simulink model "MyBattery_RTW"  (Simulink 8.5)
settings: Solver=ode1  SolverMode=SingleTasking  StartTime=0.0  StopTime=inf  FixedStep=0.0002  RelTol=1e-3
PreLoadFcn:
  | vehicle = 'Car'; if ~length(which('cmcmd')), cmenv; end
  | MyBattery_RTW_bus
InitFcn:
  | vehicle = 'Car'; if ~length(which('cmcmd')), cmenv; end
  | MyBattery_RTW_bus
libraries: CarMaker4SL x2, simulink x2
Description:
  | CarMaker Real-Time Target (64-bit)
settings Model: Creator=ml  LastModifiedBy=ml
settings DebuggingCC: FcnCallInpInsideContextMsg=UseLocalSettings
settings HardwareCC: TargetHWDeviceType=32-bit Generic  ProdEqTarget=off
settings RTWCC: SystemTargetFile=CarMaker64.tlc  TemplateMakefile=CarMaker_unix64.tmf  Description=CarMaker Real-Time Target (64-bit)
settings CodeAppCC: MaxIdLength=63
settings STFCustomTargetCC: ModelReferenceCompliant=off  GeneratePreprocessorConditionals=Disable all  MultiInstanceERTCode=on  CodeInterfacePackaging=Reusable function  CPPClassGenCompliant=on  GRTInterface=off  GenerateAllocFcn=on  SystemTargetFile=CarMaker64.tlc
settings GRTTargetCC: ModelReferenceCompliant=off  ParMdlRefBuildCompliant=off  CompOptLevelCompliant=off  ConcurrentExecutionCompliant=off  MatFileLogging=off  MultiInstanceERTCode=on  CodeInterfacePackaging=Reusable function  GRTInterface=off  GenerateAllocFcn=on  ExtModeMexFile=noextcomm
settings CustomProperty: DataType=string  Value=..
settings EnumStrPairs: String=Car

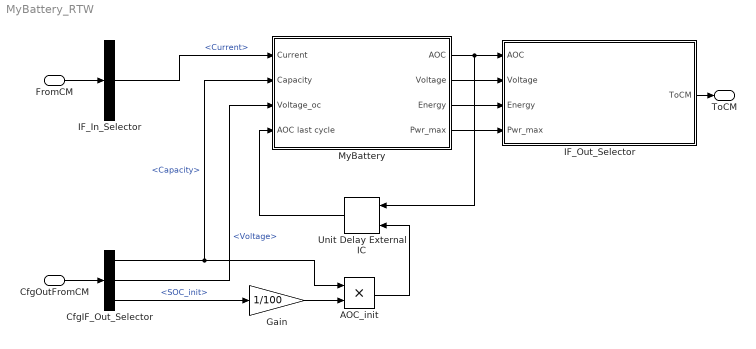
== system MyBattery_RTW ==
  FromCM : Inport  OutDataTypeStr=Bus: cmPTBatteryIn
  CfgOutFromCM : Inport  Port=2  OutDataTypeStr=Bus: cmPTBatteryCfgOut
  AOC_init : Product  RndMeth=Zero
  CfgIF_Out_Selector : BusSelector  OutputSignals=Capacity,Voltage,SOC_init
  Gain : Gain  Gain=1/100
  IF_In_Selector : BusSelector  OutputSignals=Current
  IF_Out_Selector : Subsystem  mask(Signal Selection){}
      mask help: Signal Selection Block
      settings: OpenFcn=cmSignalSelect('SignalSelection_CB',gcb)
  MyBattery : Subsystem
  Unit Delay External IC : simulink/Additional Math & Discrete/Additional Discrete/Unit Delay External IC  tsamp=-1
  ToCM : Outport  OutDataTypeStr=Bus: cmPTBatteryOut
  wires:
  FromCM/1 -> IF_In_Selector/1
  IF_Out_Selector/1(ToCM) -> ToCM/1
  CfgOutFromCM/1 -> CfgIF_Out_Selector/1
  IF_In_Selector/1 -> MyBattery/1(Current)  "<Current>"
  MyBattery/1(AOC) -> Unit Delay External IC/1, IF_Out_Selector/1(AOC)
  MyBattery/2(Voltage) -> IF_Out_Selector/2(Voltage)
  MyBattery/3(Energy) -> IF_Out_Selector/3(Energy)
  MyBattery/4(Pwr_max) -> IF_Out_Selector/4(Pwr_max)
  CfgIF_Out_Selector/1 -> MyBattery/2(Capacity), AOC_init/1  "<Capacity>"
  Unit Delay External IC/1 -> MyBattery/4(AOC last cycle)
  AOC_init/1 -> Unit Delay External IC/2
  Gain/1 -> AOC_init/2
  CfgIF_Out_Selector/3 -> Gain/1  "<SOC_init>"
  CfgIF_Out_Selector/2 -> MyBattery/3(Voltage_oc)  "<Voltage>"

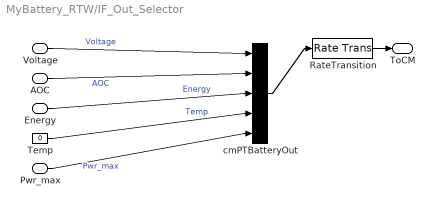
== system MyBattery_RTW/IF_Out_Selector ==
  AOC : Inport
  Voltage : Inport  Port=2
  Energy : Inport  Port=3
  Pwr_max : Inport  Port=4
  RateTransition : RateTransition  OutPortSampleTime=str2num(get_param(bdroot,'FixedStep'))
  Temp : Constant  Value=0
  cmPTBatteryOut : BusCreator  Inputs=5
  ToCM : Outport
  wires:
  RateTransition/1 -> ToCM/1
  cmPTBatteryOut/1 -> RateTransition/1
  Temp/1 -> cmPTBatteryOut/4  "Temp"
  AOC/1 -> cmPTBatteryOut/2  "AOC"
  Voltage/1 -> cmPTBatteryOut/1  "Voltage"
  Energy/1 -> cmPTBatteryOut/3  "Energy"
  Pwr_max/1 -> cmPTBatteryOut/5  "Pwr_max"

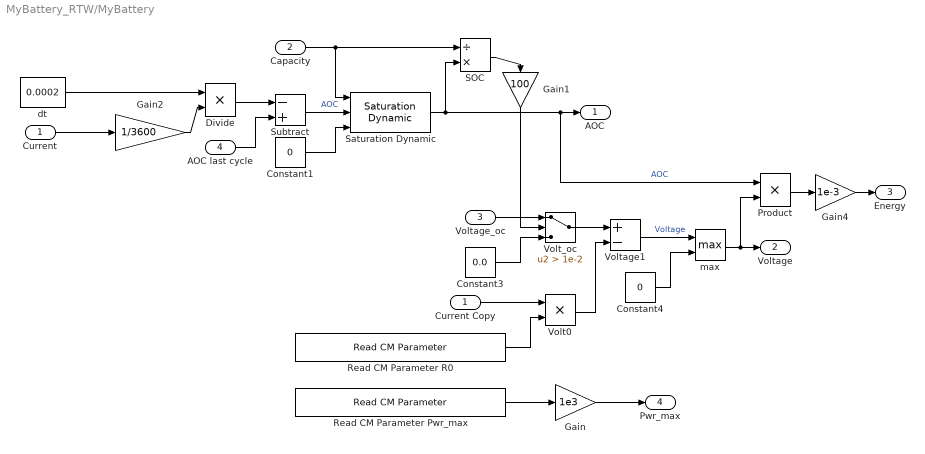
== system MyBattery_RTW/MyBattery ==
  Current : Inport
  Capacity : Inport  Port=2
  Voltage_oc : Inport  Port=3
  AOC last cycle : Inport  Port=4
  Constant1 : Constant  Value=0
  Constant3 : Constant  Value=0.0
  Constant4 : Constant  Value=0
  Current Copy : InportShadow
  Divide : Product  Inputs=**
  Gain : Gain  Gain=1e3
  Gain1 : Gain  Gain=100
  Gain2 : Gain  Gain=1/3600
  Gain4 : Gain  Gain=1e-3
  Product : Product  RndMeth=Zero
  Read CM Parameter Pwr_max : CarMaker4SL/Read CM Parameter  xfile=Vehicle  xkey=PowerTrain.PowerSupply.BattLV.Pwr_max  xnout=1  xdefaults=100  xmuxed=on
  Read CM Parameter R0 : CarMaker4SL/Read CM Parameter  xfile=Vehicle  xkey=PowerTrain.PowerSupply.BattLV.R0  xnout=1  xdefaults=0.0012  xmuxed=on
  SOC : Product  Inputs=/*
  Saturation Dynamic : simulink/Discontinuities/Saturation Dynamic  SystemSampleTime=-1  OutMin=[]  OutMax=[]  OutDataTypeStr=Inherit: Same as second input  OutDataType=sfix(16)  OutScaling=2^-10  DoSatur=off
  Subtract : Sum  Inputs=-+
  Volt0 : Product  RndMeth=Zero
  Volt_oc : Switch  Criteria=u2 > Threshold  Threshold=1e-2
  Voltage1 : Sum  Inputs=+-
  dt : Constant  Value=0.0002
  max : MinMax  Function=max  Inputs=2
  AOC : Outport
  Voltage : Outport  Port=2
  Energy : Outport  Port=3
  Pwr_max : Outport  Port=4
  wires:
  Saturation Dynamic/1 -> AOC/1, Product/1, SOC/2  "AOC"
  Divide/1 -> Subtract/1
  dt/1 -> Divide/1
  Subtract/1 -> Saturation Dynamic/2  "AOC"
  Constant1/1 -> Saturation Dynamic/3
  Capacity/1 -> Saturation Dynamic/1, SOC/1
  Read CM Parameter Pwr_max/1 -> Gain/1
  SOC/1 -> Gain1/1
  Voltage_oc/1 -> Volt_oc/1
  Constant3/1 -> Volt_oc/3
  Read CM Parameter R0/1 -> Volt0/2
  Volt_oc/1 -> Voltage1/1
  Volt0/1 -> Voltage1/2
  Voltage1/1 -> max/1  "Voltage"
  Constant4/1 -> max/2
  max/1 -> Voltage/1, Product/2
  Product/1 -> Gain4/1
  Gain/1 -> Pwr_max/1
  AOC last cycle/1 -> Subtract/2
  Gain2/1 -> Divide/2
  Gain1/1 -> Volt_oc/2
  Current/1 -> Gain2/1
  Current Copy/1 -> Volt0/1
  Gain4/1 -> Energy/1
